simulink model "HodgkinHuxley_StepResponse_unprotected"  (R2024b)
settings: Solver=VariableStepAuto  StartTime=0.0  StopTime=100.0  RelTol=1e-3
settings Model: Creator=froessil  LastModifiedBy=froessil

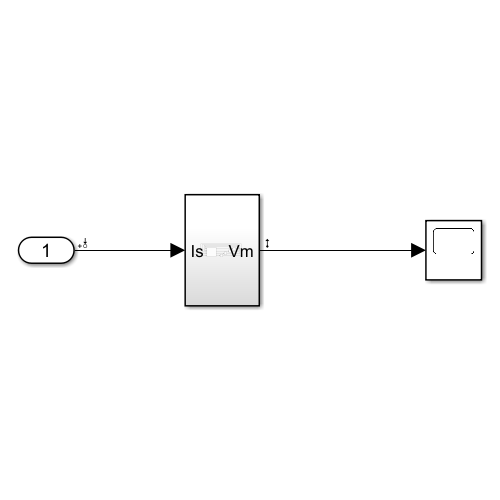
[thumbnail: Simulink's stored preview of the top-level diagram]
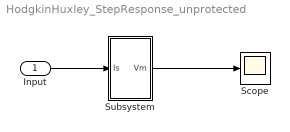
== system HodgkinHuxley_StepResponse_unprotected ==
  Input : Inport
  Scope : Scope
  Subsystem : Subsystem
  wires:
  Input/1 -> Subsystem/1(Is)
  Subsystem/1(Vm) -> Scope/1

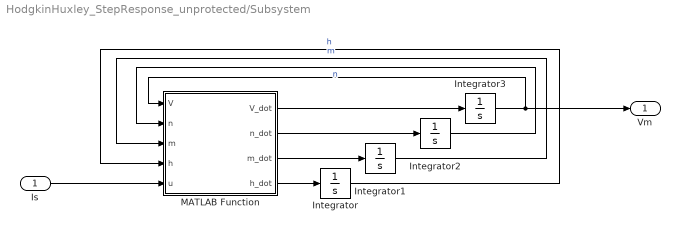
== system HodgkinHuxley_StepResponse_unprotected/Subsystem ==
  Is : Inport
  Integrator : Integrator  InitialCondition=0.595414054452739  LimitOutput=on  UpperSaturationLimit=1  LowerSaturationLimit=0
  Integrator1 : Integrator  InitialCondition=0.0529130138482760  LimitOutput=on  UpperSaturationLimit=1  LowerSaturationLimit=0
  Integrator2 : Integrator  InitialCondition=0.317563943083077  LimitOutput=on  UpperSaturationLimit=1  LowerSaturationLimit=0
  Integrator3 : Integrator  LimitOutput=on
  MATLAB Function : MATLAB Function  TreatAsAtomicUnit=on
  Vm : Outport
  wires:
  Integrator3/1 -> Vm/1, MATLAB Function/1(V)
  Integrator2/1 -> MATLAB Function/2(n)  "n"
  Integrator/1 -> MATLAB Function/4(h)  "h"
  Is/1 -> MATLAB Function/5(u)
  MATLAB Function/4(h_dot) -> Integrator/1
  Integrator1/1 -> MATLAB Function/3(m)  "m"
  MATLAB Function/2(n_dot) -> Integrator2/1
  MATLAB Function/3(m_dot) -> Integrator1/1
  MATLAB Function/1(V_dot) -> Integrator3/1

== matlab function HodgkinHuxley_StepResponse_unprotected/Subsystem/MATLAB Function ==
  data: V input; n input; m input; h input; u input; V_dot output; n_dot output; m_dot output; h_dot output
function [V_dot,n_dot,m_dot,h_dot] = neuron(V, n, m, h, u)

    Cm      = 1;    % [uF/cm2]
    g_Na    = 120;  % [mS/cm2]
    g_k     = 36;   % [mS/cm2] 
    g_l     = 0.3;  % [mS/cm2]
    V_Na    = 115;  % [mV]
    V_k     = -12;  % [mV]
    V_l     = 10.6; % [mV]

    alpha_n = 0.01*(10-V)/(exp((10-V)/10)-1);
    beta_n = 0.125*exp(-V/80);
    alpha_m = 0.1*(25-V)/(exp((25-V)/10)-1);
    beta_m = 4*exp(-V/18);
    alpha_h = 0.07*exp(-V/20);
    beta_h = 1/(exp((30-V)/10)+1);
    
    V_dot = (u/Cm) - (g_k*(n^4)*(V-V_k)/Cm) - ((m^3)*h*(V-V_Na)*g_Na/Cm) - ((g_l/Cm)*(V-V_l));

    n_dot = (alpha_n*(1-n)) - (beta_n*n);
    m_dot = (alpha_m*(1-m)) - (beta_m*m);
    h_dot = (alpha_h*(1-h)) - (beta_h*h);
    
end
